simulink model "Whole_Axle_Suspension_Model"  (R2024a)
settings: Solver=VariableStepAuto  StartTime=0.0  StopTime=10.0  FixedStep=1  RelTol=1e-3
values from neighbouring files (symbols this model uses):
  C1 = 700    [task4.m]
  C2 = 900    [task4.m]
  C3 = 300    [task4.m]
  K1 = 2200    [task4.m]
  K2 = 8000    [task4.m]
  K3 = 120000    [task4.m]
  M1 = 50    [task4.m]
  M2 = 250    [task4.m]
  M3 = 100    [task4.m]
settings Model: Creator=Rotim  LastModifiedBy=Rotim

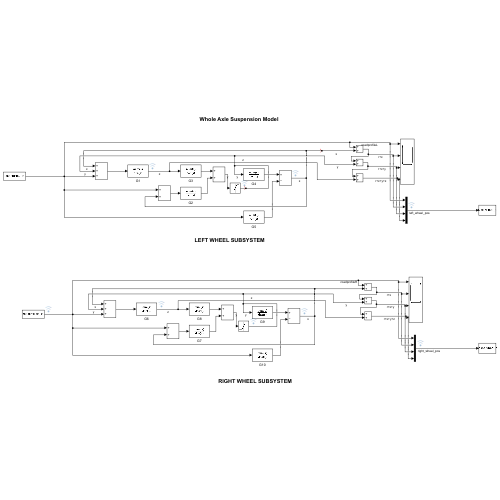
[thumbnail: Simulink's stored preview of the top-level diagram]
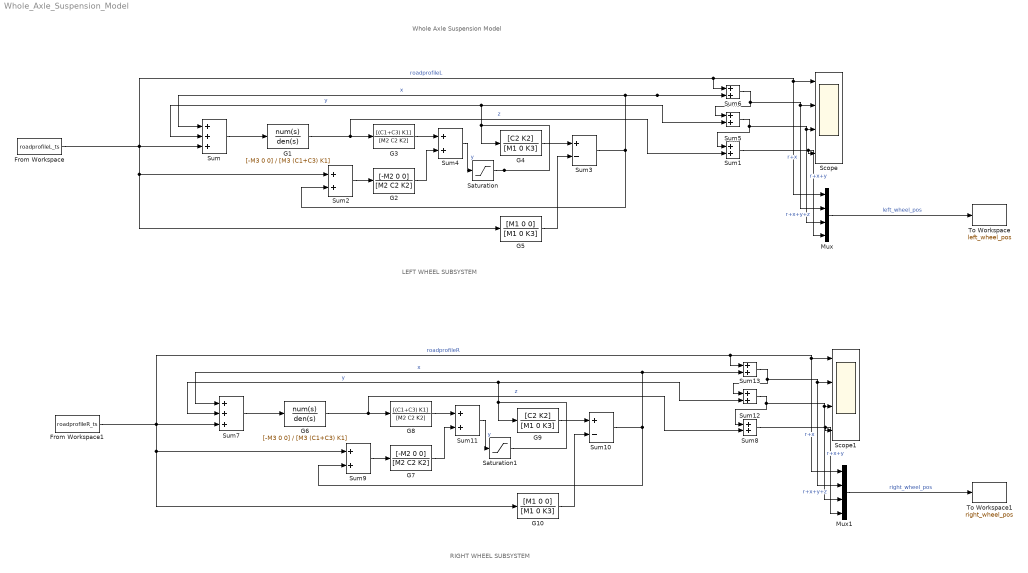
== system Whole_Axle_Suspension_Model ==
  note: Whole Axle Suspension Model
  note: LEFT WHEEL SUBSYSTEM
  note: RIGHT WHEEL SUBSYSTEM
  From Workspace : FromWorkspace  VariableName=roadprofileL_ts  SampleTime=1
  From Workspace1 : FromWorkspace  VariableName=roadprofileR_ts  SampleTime=1
  G1 : TransferFcn  Numerator=[-M3 0 0]  Denominator=[M3 (C1+C3) K1]
  G10 : TransferFcn  Numerator=[M1 0 0]  Denominator=[M1 0 K3]
  G2 : TransferFcn  Numerator=[-M2 0 0]  Denominator=[M2 C2 K2]
  G3 : TransferFcn  Numerator=[(C1+C3) K1]  Denominator=[M2 C2 K2]
  G4 : TransferFcn  Numerator=[C2 K2]  Denominator=[M1 0 K3]
  G5 : TransferFcn  Numerator=[M1 0 0]  Denominator=[M1 0 K3]
  G6 : TransferFcn  Numerator=[-M3 0 0]  Denominator=[M3 (C1+C3) K1]
  G7 : TransferFcn  Numerator=[-M2 0 0]  Denominator=[M2 C2 K2]
  G8 : TransferFcn  Numerator=[(C1+C3) K1]  Denominator=[M2 C2 K2]
  G9 : TransferFcn  Numerator=[C2 K2]  Denominator=[M1 0 K3]
  Mux : Mux
  Mux1 : Mux
  Saturation : Saturate  UpperLimit=0.02  LowerLimit=-0.02
  Saturation1 : Saturate  UpperLimit=0.02  LowerLimit=-0.02
  Scope : Scope  NumInputPorts=4
  Scope1 : Scope  NumInputPorts=4
  Sum : Sum  Inputs=+++
  Sum{1..2,4..6,8..9,11..13} (10 alike) : Sum
  Sum10 : Sum  Inputs=+-
  Sum3 : Sum  Inputs=+-
  Sum7 : Sum  Inputs=+++
  To Workspace : ToWorkspace  VariableName=left_wheel_pos  SaveFormat=Timeseries  SampleTime=-1
  To Workspace1 : ToWorkspace  VariableName=right_wheel_pos  SaveFormat=Timeseries  SampleTime=-1
  wires:
  Sum5/1 -> Sum1/1, Mux/3, Scope/3  "r+x+y"
  Mux/1 -> To Workspace/1  "left_wheel_pos"
  G2/1 -> Sum4/2
  Sum1/1 -> Mux/4, Scope/4  "r+x+y+z"
  From Workspace/1 -> Sum6/1, Mux/1, Scope/1, Sum2/1, G5/1, Sum/3  "roadprofileL"
  G3/1 -> Sum4/1
  Sum/1 -> G1/1
  Sum6/1 -> Mux/2, Scope/2, Sum5/1  "r+x"
  G1/1 -> Sum1/2, G3/1  "z"
  G5/1 -> Sum3/2
  Sum2/1 -> G2/1
  Saturation/1 -> G4/1, Sum/2, Sum5/2  "y"
  G4/1 -> Sum3/1
  Sum4/1 -> Saturation/1  "y"
  Sum3/1 -> Sum6/2, Sum/1, Sum2/2  "x"
  Sum11/1 -> Saturation1/1  "y"
  Sum10/1 -> Sum13/2, Sum7/1, Sum9/2  "x"
  G9/1 -> Sum10/1
  G10/1 -> Sum10/2
  G6/1 -> Sum8/2, G8/1  "z"
  Sum13/1 -> Mux1/2, Scope1/2, Sum12/1  "r+x"
  Sum9/1 -> G7/1
  Sum7/1 -> G6/1
  Saturation1/1 -> G9/1, Sum7/2, Sum12/2  "y"
  From Workspace1/1 -> Sum9/1, G10/1, Sum13/1, Mux1/1, Scope1/1, Sum7/3  "roadprofileR"
  G8/1 -> Sum11/1
  Sum8/1 -> Mux1/4, Scope1/4  "r+x+y+z"
  G7/1 -> Sum11/2
  Sum12/1 -> Sum8/1, Mux1/3, Scope1/3  "r+x+y"
  Mux1/1 -> To Workspace1/1  "right_wheel_pos"
